simulink library "PTOSim_Lib"  (R2021b)
settings: Solver=ode45  StartTime=0.0  StopTime=10.0  RelTol=1e-3  EnableMultiTasking=on
undefined symbols (not defined in the file or in its folder): DiscIntNeverNeededParam, PTOSimBlock, simu
libraries: $bdroot x3, simulink x2
(part 2 of 2)

== system PTOSim_Lib/Motion Conversion/Rotary to Linear Adjustable Rod/Angle Calculation for PTO/Distance btw flap joint & rod joint along x-axis ==
  Add3 : Sum  Inputs=+-
  Add4 : Sum  Inputs=+-
  Constant4 : Constant  Value=PTOSimBlock.AdjustableRod.rodInit
  Constant5 : Constant  Value=PTOSimBlock.AdjustableRod.crank
  Constant6 : Constant  Value=PTOSimBlock.AdjustableRod.offset
  Math Function2 : Math  Operator=square  SignedPower=on  SaturateOnIntegerOverflow=on
  Math Function3 : Math  Operator=square  SignedPower=on  SaturateOnIntegerOverflow=on
  Sqrt1 : Sqrt  SaturateOnIntegerOverflow=on
  d : Outport
  wires:
  Sqrt1/1 -> d/1
  Math Function2/1 -> Add3/1
  Math Function3/1 -> Add3/2
  Add4/1 -> Math Function3/1
  Constant6/1 -> Add4/2
  Constant5/1 -> Add4/1
  Constant4/1 -> Math Function2/1
  Add3/1 -> Sqrt1/1

== system PTOSim_Lib/Motion Conversion/Rotary to Linear Adjustable Rod/Angle Calculation for PTO/Subsystem1 ==
  angPos : Inport
  Add2 : Sum  Inputs=+-
  Add5 : Sum
  Add6 : Sum  Inputs=+-
  Constant1 : Constant  Value=PTOSimBlock.AdjustableRod.crank
  Constant2 : Constant  Value=PTOSimBlock.AdjustableRod.crank
  Constant3 : Constant  Value=PTOSimBlock.AdjustableRod.offset
  Distance btw flap joint & rod joint along x-axis : Subsystem
  Math Function1 : Math  Operator=square  SignedPower=on  SaturateOnIntegerOverflow=on
  Math Function6 : Math  Operator=square  SignedPower=on  SaturateOnIntegerOverflow=on
  Product1 : Product  Inputs=**
  Product7 : Product  Inputs=**
  Sqrt2 : Sqrt  SaturateOnIntegerOverflow=on
  Trigonometric Function1 : Trigonometry  Operator=cos
  Trigonometric Function5 : Trigonometry
  rodLength : Outport
  wires:
  Distance btw flap joint & rod joint along x-axis/1(d) -> Add6/1
  Constant2/1 -> Product7/1
  Math Function1/1 -> Add5/1
  Constant3/1 -> Add2/2
  Product1/1 -> Add2/1
  Trigonometric Function1/1 -> Product1/2
  Constant1/1 -> Product1/1
  Sqrt2/1 -> rodLength/1
  Add5/1 -> Sqrt2/1
  Math Function6/1 -> Add5/2
  Add6/1 -> Math Function6/1
  Product7/1 -> Add6/2
  Trigonometric Function5/1 -> Product7/2
  Add2/1 -> Math Function1/1
  angPos/1 -> Trigonometric Function1/1, Trigonometric Function5/1

== system PTOSim_Lib/Motion Conversion/Rotary to Linear Adjustable Rod/Angle Calculation for PTO/Subsystem2 ==
  angPos : Inport
  Add2 : Sum  Inputs=+-
  Add5 : Sum
  Add6 : Sum  Inputs=+-
  Constant1 : Constant  Value=PTOSimBlock.AdjustableRod.crank
  Constant2 : Constant  Value=PTOSimBlock.AdjustableRod.crank
  Constant3 : Constant  Value=PTOSimBlock.AdjustableRod.offset
  Distance btw flap joint & rod joint along x-axis : Subsystem
  Math Function1 : Math  Operator=square  SignedPower=on  SaturateOnIntegerOverflow=on
  Math Function6 : Math  Operator=square  SignedPower=on  SaturateOnIntegerOverflow=on
  Product1 : Product  Inputs=**
  Product7 : Product  Inputs=**
  Sqrt2 : Sqrt  SaturateOnIntegerOverflow=on
  Trigonometric Function1 : Trigonometry  Operator=cos
  Trigonometric Function5 : Trigonometry
  rodLength : Outport
  wires:
  Distance btw flap joint & rod joint along x-axis/1(d) -> Add6/1
  Constant2/1 -> Product7/1
  Math Function1/1 -> Add5/1
  Constant3/1 -> Add2/2
  Product1/1 -> Add2/1
  Trigonometric Function1/1 -> Product1/2
  Constant1/1 -> Product1/1
  Sqrt2/1 -> rodLength/1
  Add5/1 -> Sqrt2/1
  Math Function6/1 -> Add5/2
  Add6/1 -> Math Function6/1
  Product7/1 -> Add6/2
  Trigonometric Function5/1 -> Product7/2
  Add2/1 -> Math Function1/1
  angPos/1 -> Trigonometric Function1/1, Trigonometric Function5/1

== system PTOSim_Lib/Motion Conversion/Rotary to Linear Adjustable Rod/Angular to Linear Position/Distance btw flap joint & rod joint along x-axis ==
  Add3 : Sum  Inputs=+-
  Add4 : Sum  Inputs=+-
  Constant4 : Constant  Value=PTOSimBlock.AdjustableRod.rodInit
  Constant5 : Constant  Value=PTOSimBlock.AdjustableRod.crank
  Constant6 : Constant  Value=PTOSimBlock.AdjustableRod.offset
  Math Function2 : Math  Operator=square  SignedPower=on  SaturateOnIntegerOverflow=on
  Math Function3 : Math  Operator=square  SignedPower=on  SaturateOnIntegerOverflow=on
  Sqrt1 : Sqrt  SaturateOnIntegerOverflow=on
  d : Outport
  wires:
  Add3/1 -> Sqrt1/1
  Constant4/1 -> Math Function2/1
  Constant5/1 -> Add4/1
  Constant6/1 -> Add4/2
  Add4/1 -> Math Function3/1
  Math Function3/1 -> Add3/2
  Math Function2/1 -> Add3/1
  Sqrt1/1 -> d/1

== system PTOSim_Lib/Motion Conversion/Rotary to Linear Adjustable Rod/Angular to Linear Velocity/Distance btw flap joint & rod joint along x-axis ==
  Add3 : Sum  Inputs=+-
  Add4 : Sum  Inputs=+-
  Constant4 : Constant  Value=PTOSimBlock.AdjustableRod.rodInit
  Constant5 : Constant  Value=PTOSimBlock.AdjustableRod.crank
  Constant6 : Constant  Value=PTOSimBlock.AdjustableRod.offset
  Math Function2 : Math  Operator=square  SignedPower=on  SaturateOnIntegerOverflow=on
  Math Function3 : Math  Operator=square  SignedPower=on  SaturateOnIntegerOverflow=on
  Sqrt1 : Sqrt  SaturateOnIntegerOverflow=on
  d : Outport
  wires:
  Add3/1 -> Sqrt1/1
  Constant4/1 -> Math Function2/1
  Constant5/1 -> Add4/1
  Constant6/1 -> Add4/2
  Add4/1 -> Math Function3/1
  Math Function3/1 -> Add3/2
  Math Function2/1 -> Add3/1
  Sqrt1/1 -> d/1

== system PTOSim_Lib/Motion Conversion/Rotary to Linear Adjustable Rod/Angular to Linear Velocity/Subsystem ==
  angPos : Inport
  Add2 : Sum  Inputs=+-
  Add5 : Sum
  Add6 : Sum  Inputs=+-
  Constant2 : Constant  Value=PTOSimBlock.AdjustableRod.crank
  Constant3 : Constant  Value=PTOSimBlock.AdjustableRod.offset
  Constant7 : Constant  Value=PTOSimBlock.AdjustableRod.crank
  Distance btw flap joint & rod joint along x-axis : Subsystem
  Math Function1 : Math  Operator=square  SignedPower=on  SaturateOnIntegerOverflow=on
  Math Function6 : Math  Operator=square  SignedPower=on  SaturateOnIntegerOverflow=on
  Product1 : Product  Inputs=**
  Product7 : Product  Inputs=**
  Sqrt2 : Sqrt  SaturateOnIntegerOverflow=on
  Trigonometric Function1 : Trigonometry  Operator=cos
  Trigonometric Function5 : Trigonometry
  rodLength : Outport
  wires:
  angPos/1 -> Trigonometric Function5/1, Trigonometric Function1/1
  Add2/1 -> Math Function1/1
  Trigonometric Function5/1 -> Product7/2
  Product7/1 -> Add6/2
  Add6/1 -> Math Function6/1
  Math Function6/1 -> Add5/2
  Add5/1 -> Sqrt2/1
  Sqrt2/1 -> rodLength/1
  Constant2/1 -> Product1/1
  Trigonometric Function1/1 -> Product1/2
  Product1/1 -> Add2/1
  Constant3/1 -> Add2/2
  Math Function1/1 -> Add5/1
  Constant7/1 -> Product7/1
  Distance btw flap joint & rod joint along x-axis/1(d) -> Add6/1

== system PTOSim_Lib/Motion Conversion/Rotary to Linear Crank/Angular to Linear Position/Initial Distance btw flap joint & crank joint along x-axis ==
  Add3 : Sum  Inputs=+-
  Add4 : Sum  Inputs=+-
  Constant1 : Constant  Value=PTOSimBlock.LinearCrank.rodLength
  Constant5 : Constant  Value=PTOSimBlock.LinearCrank.crank
  Constant6 : Constant  Value=PTOSimBlock.LinearCrank.offset
  Math Function2 : Math  Operator=square  SignedPower=on  SaturateOnIntegerOverflow=on
  Math Function3 : Math  Operator=square  SignedPower=on  SaturateOnIntegerOverflow=on
  Sqrt1 : Sqrt  SaturateOnIntegerOverflow=on
  d : Outport
  wires:
  Add3/1 -> Sqrt1/1
  Constant1/1 -> Math Function2/1
  Constant5/1 -> Add4/1
  Constant6/1 -> Add4/2
  Add4/1 -> Math Function3/1
  Math Function3/1 -> Add3/2
  Math Function2/1 -> Add3/1
  Sqrt1/1 -> d/1

== system PTOSim_Lib/Motion Conversion/Rotary to Linear Adjustable Rod/Angle Calculation for PTO/Subsystem1/Distance btw flap joint & rod joint along x-axis ==
  Add3 : Sum  Inputs=+-
  Add4 : Sum  Inputs=+-
  Constant1 : Constant  Value=PTOSimBlock.AdjustableRod.crank
  Constant2 : Constant  Value=PTOSimBlock.AdjustableRod.rodInit
  Constant3 : Constant  Value=PTOSimBlock.AdjustableRod.offset
  Math Function2 : Math  Operator=square  SignedPower=on  SaturateOnIntegerOverflow=on
  Math Function3 : Math  Operator=square  SignedPower=on  SaturateOnIntegerOverflow=on
  Sqrt1 : Sqrt  SaturateOnIntegerOverflow=on
  d : Outport
  wires:
  Sqrt1/1 -> d/1
  Math Function2/1 -> Add3/1
  Math Function3/1 -> Add3/2
  Add4/1 -> Math Function3/1
  Constant3/1 -> Add4/2
  Constant1/1 -> Add4/1
  Constant2/1 -> Math Function2/1
  Add3/1 -> Sqrt1/1

== system PTOSim_Lib/Motion Conversion/Rotary to Linear Adjustable Rod/Angle Calculation for PTO/Subsystem2/Distance btw flap joint & rod joint along x-axis ==
  Add3 : Sum  Inputs=+-
  Add4 : Sum  Inputs=+-
  Constant1 : Constant  Value=PTOSimBlock.AdjustableRod.crank
  Constant2 : Constant  Value=PTOSimBlock.AdjustableRod.rodInit
  Constant3 : Constant  Value=PTOSimBlock.AdjustableRod.offset
  Math Function2 : Math  Operator=square  SignedPower=on  SaturateOnIntegerOverflow=on
  Math Function3 : Math  Operator=square  SignedPower=on  SaturateOnIntegerOverflow=on
  Sqrt1 : Sqrt  SaturateOnIntegerOverflow=on
  d : Outport
  wires:
  Sqrt1/1 -> d/1
  Math Function2/1 -> Add3/1
  Math Function3/1 -> Add3/2
  Add4/1 -> Math Function3/1
  Constant3/1 -> Add4/2
  Constant1/1 -> Add4/1
  Constant2/1 -> Math Function2/1
  Add3/1 -> Sqrt1/1

== system PTOSim_Lib/Motion Conversion/Rotary to Linear Adjustable Rod/Angular to Linear Velocity/Subsystem/Distance btw flap joint & rod joint along x-axis ==
  Add3 : Sum  Inputs=+-
  Add4 : Sum  Inputs=+-
  Constant4 : Constant  Value=PTOSimBlock.AdjustableRod.rodInit
  Constant5 : Constant  Value=PTOSimBlock.AdjustableRod.crank
  Constant6 : Constant  Value=PTOSimBlock.AdjustableRod.offset
  Math Function2 : Math  Operator=square  SignedPower=on  SaturateOnIntegerOverflow=on
  Math Function3 : Math  Operator=square  SignedPower=on  SaturateOnIntegerOverflow=on
  Sqrt1 : Sqrt  SaturateOnIntegerOverflow=on
  d : Outport
  wires:
  Add3/1 -> Sqrt1/1
  Constant4/1 -> Math Function2/1
  Constant5/1 -> Add4/1
  Constant6/1 -> Add4/2
  Add4/1 -> Math Function3/1
  Math Function3/1 -> Add3/2
  Math Function2/1 -> Add3/1
  Sqrt1/1 -> d/1
